simulink model "Project4"  (R2024a)
settings: Solver=VariableStepAuto  StartTime=0.0  StopTime=10.0  MaxStep=0.05  RelTol=1e-3
values from neighbouring files (symbols this model uses):
  b = 3.5077E-6    (= 3.5077e-06)    [Project10Mscript.m]    (also in Project3Mscript.m = 2; Project4Mscript.m = 0; Project7Mscript.m = 10)
  F = 1    [Project3Mscript.m]    (also in Project4Mscript.m; Project7Mscript.m; Project_2Mscript.m = 5)
  k = 20    [Project3Mscript.m]    (also in Project4Mscript.m; Project7Mscript.m)
  M = 1    [Project3Mscript.m]    (also in Project4Mscript.m; Project7Mscript.m)
settings Model: Creator=harsh  LastModifiedBy=harsh

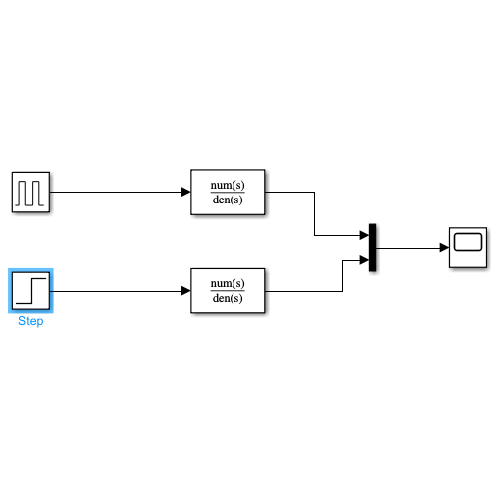
[thumbnail: Simulink's stored preview of the top-level diagram]
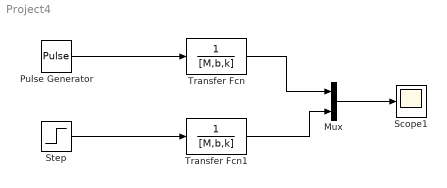
== system Project4 ==
  Mux : Mux  Inputs=2
  Pulse Generator : DiscretePulseGenerator  PulseType=Time based  Amplitude=10  Period=10  PulseWidth=5
  Scope1 : Scope
  Step : Step  After=F  SampleTime=0
  Transfer Fcn : TransferFcn  Denominator=[M,b,k]
  Transfer Fcn1 : TransferFcn  Denominator=[M,b,k]
  wires:
  Pulse Generator/1 -> Transfer Fcn/1
  Transfer Fcn/1 -> Mux/1
  Transfer Fcn1/1 -> Mux/2
  Mux/1 -> Scope1/1
  Step/1 -> Transfer Fcn1/1
